simulink model "System_Model_Hall_switch"  (Simulink 7.6)
settings: Solver=ode15s  StartTime=0.0  StopTime=3  RelTol=1e-3
undefined symbols (not defined in the file): C, g, L0, m, magnitude, Q, R, Ts, x01, x02, x03
CloseFcn:
  | rtwprivate ssgencode ModelCloseRequest System_Model1
settings Model: Creator=Fodi  LastModifiedBy=Fodi

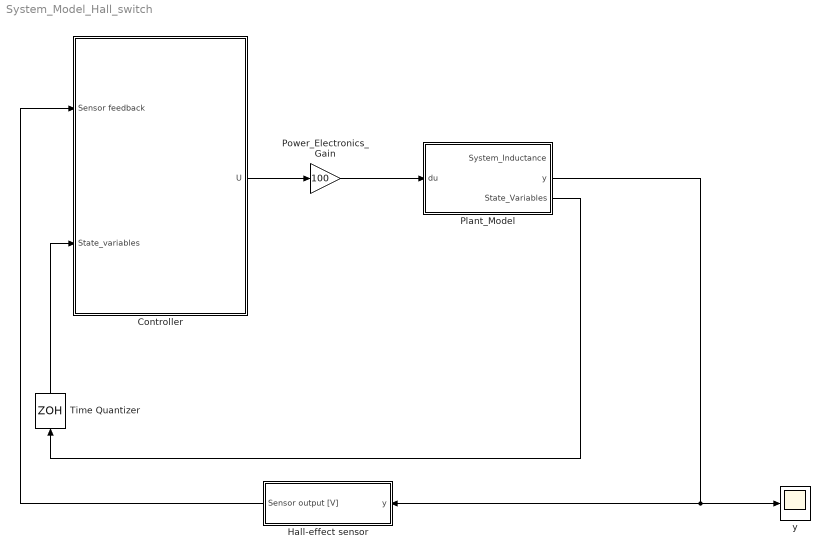
== system System_Model_Hall_switch ==
  Controller : Subsystem  TreatAsAtomicUnit=on  SystemSampleTime=Ts
  Hall-effect sensor : Subsystem
  Plant_Model : Subsystem
  Power_Electronics_Gain : Gain  Gain=100
  Time Quantizer : ZeroOrderHold  SampleTime=Ts
  y : Scope
      settings: TimeRange=3  YMin=-0.175  YMax=0.1  SaveName=y1
  wires:
  Power_Electronics_Gain/1 -> Plant_Model/1(du)
  Plant_Model/3(State_Variables) -> Time Quantizer/1
  Time Quantizer/1 -> Controller/2(State_variables)
  Controller/1(U) -> Power_Electronics_Gain/1
  Hall-effect sensor/1(Sensor output [V]) -> Controller/1(Sensor feedback)
  Plant_Model/2(y) -> Hall-effect sensor/1(y), y/1

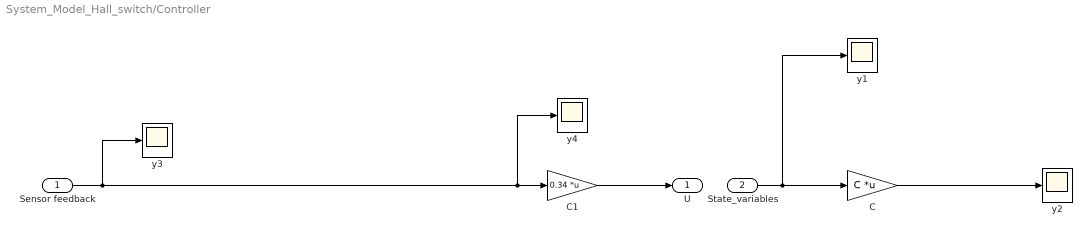
== system System_Model_Hall_switch/Controller ==
  Sensor feedback : Inport
  State_variables : Inport  Port=2
  C : Gain  Gain=C  Multiplication=Matrix(K*u)
  C1 : Gain  Gain=0.34  Multiplication=Matrix(K*u)
  y{1..4} (4 alike) : Scope
      y1 settings: TimeRange=0.3052807240566879  YMin=0.03939399134016944  YMax=0.04922765976378121  SaveName=y2
      y2 settings: TimeRange=3  YMin=-0.175  YMax=0.1  SaveName=y
      y3 settings: TimeRange=3  YMin=-0.175  YMax=0.1  SaveName=y3
      y4 settings: TimeRange=3  YMin=-0.175  YMax=0.1  SaveName=y4
  U : Outport
  wires:
  State_variables/1 -> C/1, y1/1
  C/1 -> y2/1
  Sensor feedback/1 -> y3/1, y4/1, C1/1
  C1/1 -> U/1

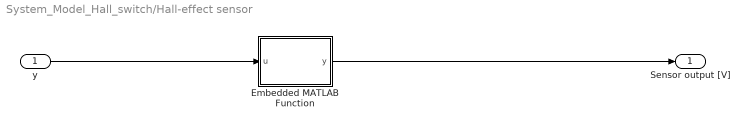
== system System_Model_Hall_switch/Hall-effect sensor ==
  y : Inport
  Embedded MATLAB Function : Stateflow chart  TreatAsAtomicUnit=on
  Sensor output [V] : Outport
  wires:
  y/1 -> Embedded MATLAB Function/1(u)
  Embedded MATLAB Function/1(y) -> Sensor output [V]/1

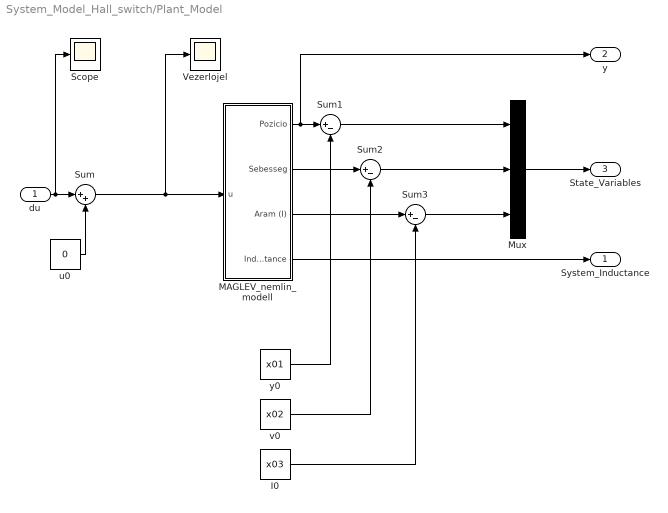
== system System_Model_Hall_switch/Plant_Model ==
  du : Inport
  I0 : Constant  Value=x03
  MAGLEV_nemlin_modell : Subsystem
  Mux : Mux  Inputs=3
  Scope : Scope
  Sum : Sum  Inputs=|++
  Sum1 : Sum  Inputs=|+-
  Sum2 : Sum  Inputs=|+-
  Sum3 : Sum  Inputs=|+-
  Vezerlojel : Scope
      settings: TimeRange=10  YMin=11  YMax=16
  u0 : Constant  Value=0
  v0 : Constant  Value=x02
  y0 : Constant  Value=x01
  System_Inductance : Outport
  y : Outport  Port=2
  State_Variables : Outport  Port=3
  wires:
  y0/1 -> Sum1/2
  v0/1 -> Sum2/2
  I0/1 -> Sum3/2
  MAGLEV_nemlin_modell/3(Aram (I)) -> Sum3/1
  Sum3/1 -> Mux/3
  Sum2/1 -> Mux/2
  Sum1/1 -> Mux/1
  u0/1 -> Sum/2
  Mux/1 -> State_Variables/1
  MAGLEV_nemlin_modell/2(Sebesseg) -> Sum2/1
  MAGLEV_nemlin_modell/1(Pozicio) -> Sum1/1, y/1
  du/1 -> Scope/1, Sum/1
  Sum/1 -> MAGLEV_nemlin_modell/1(u), Vezerlojel/1
  MAGLEV_nemlin_modell/4(Inductance) -> System_Inductance/1

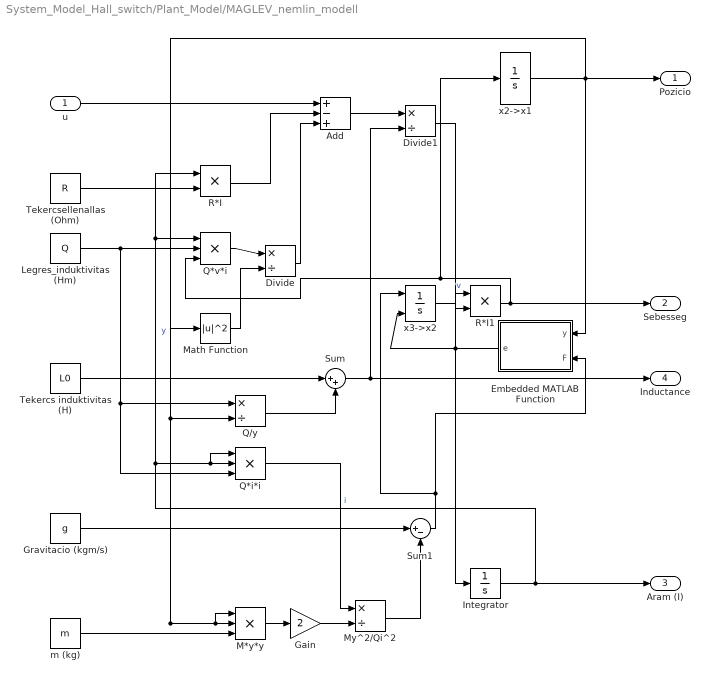
== system System_Model_Hall_switch/Plant_Model/MAGLEV_nemlin_modell ==
  u : Inport  Tag=v
  Add : Sum  Inputs=+-+
  Divide : Product  Inputs=*/
  Divide1 : Product  Inputs=*/
  Embedded MATLAB Function : Stateflow chart  TreatAsAtomicUnit=on
  Gain : Gain  Gain=2
  Gravitacio (kgm/s) : Constant  Value=g
  Integrator : Integrator  LimitOutput=on  LowerSaturationLimit=0  ContinuousStateAttributes='current'
  Legres_induktivitas (Hm) : Constant  Value=Q
  M*y*y : Product  Inputs=3  RndMeth=Zero
  Math Function : Math  Operator=magnitude^2  SaturateOnIntegerOverflow=on
  My^2/Qi^2 : Product  Inputs=*/
  Q*i*i : Product  Inputs=3  RndMeth=Zero
  Q*v*i : Product  Inputs=3  RndMeth=Zero
  Q/y : Product  Inputs=*/
  R*I : Product  RndMeth=Zero
  R*I1 : Product  RndMeth=Zero
  Sum : Sum  Inputs=|++
  Sum1 : Sum  Inputs=|+-
  Tekercs induktivitas (H) : Constant  Value=L0
  Tekercsellenallas (Ohm) : Constant  Value=R
  m (kg) : Constant  Value=m
  x2->x1 : Integrator  InitialCondition=0.05  LimitOutput=on  LowerSaturationLimit=0.001  ContinuousStateAttributes='position'
  x3->x2 : Integrator  ExternalReset=rising  ContinuousStateAttributes='speed'
  Pozicio : Outport
  Sebesseg : Outport  Port=2
  Aram (I) : Outport  Port=3
  Inductance : Outport  Port=4
  wires:
  x2->x1/1 -> Q/y/2, Math Function/1, M*y*y/2, M*y*y/1, Pozicio/1, Embedded MATLAB Function/1(y)  "y"
  Gravitacio (kgm/s)/1 -> Sum1/1
  My^2/Qi^2/1 -> Sum1/2
  Gain/1 -> My^2/Qi^2/2
  M*y*y/1 -> Gain/1
  Sum/1 -> Divide1/2, Inductance/1
  Tekercs induktivitas (H)/1 -> Sum/1
  Q/y/1 -> Sum/2
  Math Function/1 -> Divide/2
  Divide/1 -> Add/3
  Q*v*i/1 -> Divide/1
  R*I/1 -> Add/2
  Divide1/1 -> Integrator/1
  Add/1 -> Divide1/1
  u/1 -> Add/1
  m (kg)/1 -> M*y*y/3
  Legres_induktivitas (Hm)/1 -> Q*v*i/2, Q/y/1, Q*i*i/3
  Tekercsellenallas (Ohm)/1 -> R*I/2
  Q*i*i/1 -> My^2/Qi^2/1
  Integrator/1 -> Aram (I)/1, Q*i*i/2, Q*i*i/1, Q*v*i/1, R*I/1  "i"
  Sum1/1 -> x3->x2/1, Embedded MATLAB Function/2(F)
  Embedded MATLAB Function/1(e) -> x3->x2/2, R*I1/2
  R*I1/1 -> Q*v*i/3, x2->x1/1, Sebesseg/1
  x3->x2/1 -> R*I1/1  "v"

== matlab function Hall-effect sensor/Embedded MATLAB Function ==
  data: u input double; y output double
function y = fcn(u)

if (u > 0.05)
    y = 1;
else
    y = 0;
end
end

== matlab function Plant_Model/MAGLEV_nemlin_modell/Embedded MATLAB Function ==
  data: y input double; F input double; e output double
function e = fcn(y, F)
%#eml

if (F<=0 && y == 0.001)
    e=0;
else
    e=1;
end

end
